simulink library "lib_accessory"  (Simulink 4.1.1)
undefined symbols (not defined in the file): acc_dcdc_eff, acc_elec_eff, acc_elec_efficiency, acc_elec_pwr, acc_mech_eff, acc_mech_pwr, acc_mech_trq, acc_sindafile, amb_tmp, cyc_mph, ess_on, fc_on, fd_ratio, gb_ratio, load_on, map_spd, max_pwr, tc_gc_to_fc_ratio, time_step, vc_idle_bool, vc_idle_spd, vinf, wh_radius
libraries: lib_accessory x47, lib_cosimulation x29, lib_outputs x11, simulink3 x4, sub_lib_models x2
(part 1 of 3)
settings Model: LastModifiedBy=abrooker  ModifiedComment=abrooker -- Fri Jun 21 11:06:39 2002 -- Version 1.443
settings Model: ModifiedHistory=|
  | abrooker -- Fri Jun 21 11:06:39 2002 -- Version 1.443
  | 
  | 
  | abrooker -- Fri Jun 21 11:06:32 2002 -- Version 1.442
  | 
  | 
  | abrooker -- Fri Jun 21 11:03:06 2002 -- Version 1.441
  | 
  | 
  | abrooker -- Fri Jun 21 08:18:53 2002 -- Version 1.440
  | 
  | 
  | abrooker -- Fri Jun 21 08:07:14 2002 -- Version 1.439
  | 
  | 
  | abrooker -- Fri Jun 21 07:53:07 2002 -- Version 1.438
  | 
  | 
  | abrooker -- Thu Jun 20 15:33:10 2002 -- Version 1.437
  | 
  | 
  | abrooker -- Thu Jun 20 15:32:18 2002 -- Version 1.436
  | 
  | 
  | mokeefe -- Wed May 22 16:23:29 2002 -- Version 1.435
  | changed SindaTransAC model to take 5 outputs
  | 
  | mokeefe -- Thu Apr 18 08:24:09 2002 -- Version 1.434
  | saving the model:
  | o "without the model browser open"
  | o with only top-level screen visible
  | o with "fit to view" enabled
  | o with "status bar" off and "toolbar" off
  | o with "prompt to update model history with each save" on
  | 
  | tmarkel -- Mon Apr 15 11:38:46 2002 -- Version 1.428
  | 
  | 
  | tmarkel -- Mon Apr 15 11:38:46 2002 -- Version 1.428
  | 
  | 
  | tmarkel -- Mon Apr 15 11:38:36 2002 -- Version 1.427
  | 
  | 
  | mokeefe -- Mon Apr 15 11:36:55 2002 -- Version 1.426
  | added acc_sindafile variable into the SindaTransAC model
  | 
  | 
  | 
  | 
  | 
  | mokeefe -- Mon Apr 15 11:30:03 2002 -- Version 1.424
  | adding a feature to the sinda fluint s-function so that user can pass in the path to their executable file (*.im) function
  | 
  | 
  | abrooker -- Thu Apr 11 17:26:32 2002 -- Version 1.423
  | added vc_idle_bool in minimum fc shaft speed for stop/start:  otherwise
  | 
  | mokeefe -- Wed Apr 03 17:17:08 2002 -- Version 1.422
  | checked the configurable sub-system option for SindaTransAC
  | 
  | abrooker -- Tue Apr 02 08:21:35 2002 -- Version 1.421
  | 
  | 
  | abrooker -- Tue Apr 02 08:16:39 2002 -- Version 1.420
  | 
  | 
  | mokeefe -- Fri Mar 29 16:21:02 2002 -- Version 1.419
  | 
  | 
  | mokeefe -- Fri Mar 29 16:18:34 2002 -- Version 1.418
  | added SindaTransAC Sinda/Fluint cosim aux. model (transient air condition modeling)
  | 
  | mokeefe -- Fri Mar 29 09:01:44 2002 -- Version 1.417
  | 
  | 
  | mokeefe -- Fri Mar 29 09:00:29 2002 -- Version 1.416
  | 
  | 
  | mokeefe -- Fri Mar 29 08:55:21 2002 -- Version 1.415
  | 
  | 
  | mokeefe -- Fri Mar 29 08:54:32 2002 -- Version 1.414
  | 
  | 
  | mokeefe -- Fri Mar 29 08:34:07 2002 -- Version 1.413
  | 
  | 
  | mokeefe -- Fri Mar 29 08:33:22 2002 -- Version 1.412
  | rearranging the library for aesthetic purposes =)
  | 
  | mokeefe -- Fri Mar 29 08:27:44 2002 -- Version 1.411
  | took out two of the mechanical accessory options that will probably not be used (the same functionality is available with the remaining blocks). These blocks moved to the development subsystem for storage.
  | 
  | abrooker -- Thu Mar 28 16:18:46 2002 -- Version 1.410
  | (mokeefe) changed the Mechanical Accessory Load Driveline Block to use memory blocks for torque and power estimation (as opposed to two calculations)
  | 
  | abrooker -- Thu Mar 28 12:33:24 2002 -- Version 1.409
  | 
  | 
  | abrooker -- Thu Mar 28 12:25:41 2002 -- Version 1.408
  | 
  | 
  | abrooker -- Thu Mar 28 12:08:36 2002 -- Version 1.407
  | 
  | 
  | abrooker -- Thu Mar 28 12:04:18 2002 -- Version 1.406
  | 
  | 
  | abrooker -- Thu Mar 28 08:53:24 2002 -- Version 1.405
  | 
  | 
  | abrooker -- Thu Mar 28 08:49:44 2002 -- Version 1.404
  | 
  | 
  | mokeefe -- Wed Mar 27 07:38:24 2002 -- Version 1.403
  | 
  | 
  | mokeefe -- Wed Mar 27 07:37:49 2002 -- Version 1.402
  | added a masked variable (acc_max_spd) to the mechanical accessory loads library
  | 
  | mokeefe -- Wed Mar 20 10:22:56 2002 -- Version 1.401
  | changed the pictures for the configurable subsystem blocks to differentiate from the driveline blocks
  | 
  | mokeefe -- Tue Mar 12 13:44:43 2002 -- Version 1.400
  | 
  | 
  | mokeefe -- Tue Mar 12 13:36:01 2002 -- Version 1.399
  | cleaned up the library and reorganized block positions
  | 
  | 
  | mokeefe -- Tue Mar 12 13:34:33 2002 -- Version 1.398
  | 
  | 
  | mokeefe -- Tue Mar 12 13:34:15 2002 -- Version 1.397
  | 
  | 
  | mokeefe -- Tue Mar 12 13:29:31 2002 -- Version 1.396
  | 
  | 
  | mokeefe -- Tue Mar 12 13:25:46 2002 -- Version 1.395
  | 
  | 
  | mokeefe -- Tue Mar 12 13:09:55 2002 -- Version 1.394
  | changed the variable mechanical loads to include a water pump
  | 
  | mokeefe -- Tue Mar 12 12:07:07 2002 -- Version 1.393
  | 
  | 
  | mokeefe -- Tue Mar 12 12:06:03 2002 -- Version 1.392
  | 
  | 
  | mokeefe -- Tue Mar 12 12:04:31 2002 -- Version 1.391
  | 
  | 
  | mokeefe -- Tue Mar 12 11:59:22 2002 -- Version 1.390
  | 
  | 
  | mokeefe -- Tue Mar 12 11:54:25 2002 -- Version 1.389
  | changing the way that data signals are recorded (especially for the variable mechanical loads blocks--see SubLibraries/variable mechanical load --simulink implementation--)
  | 
  | mokeefe -- Fri Mar 08 07:13:02 2002 -- Version 1.388
  | added the tag acc_mech_pwr_est as a global tag to Mechanical Accessory Loads v2 <acc>
  | 
  | mokeefe -- Mon Mar 04 07:28:37 2002 -- Version 1.387
  | 
  | 
  | mokeefe -- Mon Mar 04 07:27:09 2002 -- Version 1.386
  | 
  | 
  | mokeefe -- Mon Mar 04 07:24:49 2002 -- Version 1.385
  | changed the mechanical accessory torque back to a simple version
  | 
  | mokeefe -- Fri Mar 01 16:40:21 2002 -- Version 1.384
  | 
  | 
  | mokeefe -- Fri Mar 01 16:37:19 2002 -- Version 1.383
  | 
  | 
  | mokeefe -- Fri Mar 01 15:08:33 2002 -- Version 1.382
  | 
  | 
  | mokeefe -- Fri Mar 01 12:12:06 2002 -- Version 1.381
  | 
  | 
  | mokeefe -- Fri Mar 01 12:10:27 2002 -- Version 1.380
  | 
  | 
  | mokeefe -- Fri Mar 01 11:39:14 2002 -- Version 1.379
  | 
  | 
  | mokeefe -- Fri Mar 01 11:20:41 2002 -- Version 1.378
  | 
  | 
  | mokeefe -- Fri Mar 01 10:50:57 2002 -- Version 1.377
  | 
  | 
  | mokeefe -- Fri Mar 01 10:18:24 2002 -- Version 1.376
  | 
  | 
  | mokeefe -- Fri Mar 01 10:16:01 2002 -- Version 1.375
  | 
  | 
  | mokeefe -- Fri Mar 01 10:13:39 2002 -- Version 1.374
  | 
  | 
  | mokeefe -- Fri Mar 01 09:58:45 2002 -- Version 1.373
  | 
  | 
  | mokeefe -- Fri Mar 01 09:31:13 2002 -- Version 1.372
  | 
  | 
  | mokeefe -- Fri Mar 01 09:30:34 2002 -- Version 1.371
  | 
  | 
  | mokeefe -- Fri Mar 01 09:00:19 2002 -- Version 1.370
  | 
  | 
  | mokeefe -- Fri Mar 01 08:27:00 2002 -- Version 1.369
  | 
  | 
  | mokeefe -- Fri Mar 01 08:04:14 2002 -- Version 1.368
  | 
  | 
  | mokeefe -- Thu Feb 28 08:51:52 2002 -- Version 1.367
  | 
  | 
  | mokeefe -- Thu Feb 28 08:48:14 2002 -- Version 1.366
  | 
  | 
  | mokeefe -- Thu Feb 28 08:21:55 2002 -- Version 1.365
  | 
  | 
  | mokeefe -- Thu Feb 28 08:20:46 2002 -- Version 1.364
  | adding an on/off flag for auxiliary systems to account for "engine off" states
  | 
  | mokeefe -- Thu Feb 28 08:10:24 2002 -- Version 1.363
  | 
  | 
  | mokeefe -- Wed Feb 27 14:38:39 2002 -- Version 1.362
  | 
  | 
  | mokeefe -- Wed Feb 27 14:34:06 2002 -- Version 1.361
  | 
  | 
  | mokeefe -- Wed Feb 27 14:33:33 2002 -- Version 1.360
  | 
  | 
  | mokeefe -- Wed Feb 27 14:29:19 2002 -- Version 1.359
  | 
  | 
  | mokeefe -- Wed Feb 27 14:12:33 2002 -- Version 1.358
  | 
  | 
  | mokeefe -- Wed Feb 27 14:11:56 2002 -- Version 1.357
  | 
  | 
  | mokeefe -- Wed Feb 27 14:06:17 2002 -- Version 1.356
  | 
  | 
  | mokeefe -- Wed Feb 27 14:04:01 2002 -- Version 1.355
  | added a "version 2" to mechanical auxiliary loads library which has a workaround that takes in the fc_spd_est instead of fc_spd_out_a--this enables vehicles to have an exact match between ADVISOR v3.2 and v2002
  | 
  | mokeefe -- Wed Feb 27 09:55:44 2002 -- Version 1.354
  | 
  | 
  | mokeefe -- Wed Feb 27 09:53:42 2002 -- Version 1.
  | 
  | mokeefe -- Tue Feb 26 15:16:41 2002 -- Version 1.352
  | 
  | 
  | mokeefe -- Tue Feb 26 14:01:11 2002 -- Version 1.351
  | 
  | 
  | mokeefe -- Tue Feb 26 13:25:47 2002 -- Version 1.350
  | 
  | 
  | mokeefe -- Tue Feb 26 10:40:53 2002 -- Version 1.349
  | 
  | 
  | mokeefe -- Mon Feb 25 16:05:53 2002 -- Version 1.348
  | 
  | 
  | mokeefe -- Mon Feb 25 15:35:04 2002 -- Version 1.347
  | 
  | 
  | mokeefe -- Mon Feb 25 15:33:00 2002 -- Version 1.346
  | 
  | 
  | mokeefe -- Mon Feb 25 15:26:23 2002 -- Version 1.345
  | 
  | 
  | mokeefe -- Mon Feb 25 15:24:36 2002 -- Version 1.344
  | 
  | 
  | mokeefe -- Mon Feb 25 15:23:19 2002 -- Version 1.343
  | 
  | 
  | mokeefe -- Mon Feb 25 15:19:58 2002 -- Version 1.342
  | 
  | 
  | mokeefe -- Mon Feb 25 15:17:22 2002 -- Version 1.341
  | 
  | 
  | mokeefe -- Mon Feb 25 15:04:08 2002 -- Version 1.340
  | 
  | 
  | mokeefe -- Mon Feb 25 14:59:43 2002 -- Version 1.339
  | 
  | 
  | mokeefe -- Mon Feb 25 14:50:11 2002 -- Version 1.338
  | 
  | 
  | mokeefe -- Mon Feb 25 14:37:23 2002 -- Version 1.337
  | 
  | 
  | mokeefe -- Mon Feb 25 14:24:02 2002 -- Version 1.336
  | 
  | 
  | mokeefe -- Mon Feb 25 14:19:40 2002 -- Version 1.335
  | 
  | 
  | mokeefe -- Mon Feb 25 14:14:18 2002 -- Version 1.334
  | 
  | 
  | mokeefe -- Mon Feb 25 14:09:13 2002 -- Version 1.333
  | 
  | 
  | mokeefe -- Mon Feb 25 13:38:54 2002 -- Version 1.332
  | 
  | 
  | mokeefe -- Mon Feb 25 13:38:02 2002 -- Version 1.331
  | 
  | 
  | mokeefe -- Wed Feb 20 09:52:02 2002 -- Version 1.330
  | 
  | 
  | mokeefe -- Wed Feb 20 09:49:29 2002 -- Version 1.329
  | changed the acc_mech_trq_a, acc_mech_pwr_a, acc_mech_trq_r, acc_mech_pwr_r, acc_elec_pwr_a, acc_elec_pwr_r GOTO blocks to global scope.
  | 
  | mokeefe -- Wed Feb 20 09:47:28 2002 -- Version 1.328
  | 
  | 
  | mokeefe -- Wed Feb 20 09:46:46 2002 -- Version 1.327
  | 
  | 
  | mokeefe -- Wed Feb 20 07:42:37 2002 -- Version 1.326
  | 
  | 
  | mokeefe -- Wed Feb 20 07:42:12 2002 -- Version 1.325
  | 
  | 
  | mokeefe -- Wed Feb 20 07:41:46 2002 -- Version 1.324
  | 
  | 
  | mokeefe -- Tue Feb 19 16:34:31 2002 -- Version 1.323
  | 
  | 
  | mokeefe -- Tue Feb 19 16:31:37 2002 -- Version 1.322
  | 
  | 
  | mokeefe -- Tue Feb 19 16:28:38 2002 -- Version 1.321
  | changed the accessory GOTO tags to global scope in Electrical Accessory Loads
  | 
  | mokeefe -- Tue Feb 19 16:14:33 2002 -- Version 1.320
  | first release to RCS
  | 
  | mokeefe -- Tue Feb 19 16:12:28 2002 -- Version 1.319
  | 
  | 
  | mokeefe -- Tue Feb 19 16:06:11 2002 -- Version 1.318
  | 
  | 
  | mokeefe -- Tue Feb 19 16:02:32 2002 -- Version 1.317
  | 
  | 
  | mokeefe -- Tue Feb 19 15:58:43 2002 -- Version 1.316
  | 
  | 
  | mokeefe -- Tue Feb 19 15:55:41 2002 -- Version 1.315
  | 
  | 
  | mokeefe -- Tue Feb 19 15:53:46 2002 -- Version 1.314
  | 
  | 
  | mokeefe -- Tue Feb 19 15:49:12 2002 -- Version 1.313
  | 
  | 
  | mokeefe -- Tue Feb 19 15:42:48 2002 -- Version 1.312
  | 
  | 
  | mokeefe -- Tue Feb 19 15:41:05 2002 -- Version 1.311
  | 
  | 
  | mokeefe -- Tue Feb 19 15:38:40 2002 -- Version 1.310
  | 
  | 
  | mokeefe -- Tue Feb 19 15:28:06 2002 -- Version 1.309
  | 
  | 
  | mokeefe -- Tue Feb 19 15:18:02 2002 -- Version 1.308
  | 
  | 
  | mokeefe -- Tue Feb 19 14:53:21 2002 -- Version 1.307
  | 
  | 
  | mokeefe -- Tue Feb 19 14:46:24 2002 -- Version 1.306
  | 
  | 
  | mokeefe -- Tue Feb 19 14:20:08 2002 -- Version 1.305
  | 
  | 
  | mokeefe -- Tue Feb 19 14:15:36 2002 -- Version 1.304
  | 
  | 
  | mokeefe -- Tue Feb 19 13:24:42 2002 -- Version 1.303
  | 
  | 
  | mokeefe -- Tue Feb 19 13:17:05 2002 -- Version 1.302
  | 
  | 
  | mokeefe -- Tue Feb 19 13:11:20 2002 -- Version 1.301
  | 
  | 
  | mokeefe -- Tue Feb 19 11:29:38 2002 -- Version 1.300
  | 
  | 
  | mokeefe -- Tue Feb 19 11:24:45 2002 -- Version 1.299
  | adding electrical accessory block
  | 
  | 
  | mokeefe -- Tue Feb 19 10:53:36 2002 -- Version 1.298
  | 
  | 
  | mokeefe -- Tue Feb 19 10:19:54 2002 -- Version 1.297
  | added electrical accessory loads block
  | 
  | 
  | mokeefe -- Thu Feb 14 17:56:03 2002 -- Version 1.296
  | 
  | 
  | mokeefe -- Thu Feb 14 17:54:33 2002 -- Version 1.295
  | 
  | 
  | mokeefe -- Thu Feb 14 17:51:07 2002 -- Version 1.294
  | 
  | 
  | mokeefe -- Thu Feb 14 17:49:19 2002 -- Version 1.293
  | changing the way that data is "logged" to displays and scopes vs. workspace on some components that I expect will have to be used multiple times... (a workaround for now)
  | 
  | mokeefe -- Thu Feb 14 17:21:35 2002 -- Version 1.292
  | 
  | 
  | mokeefe -- Thu Feb 14 16:55:33 2002 -- Version 1.291
  | 
  | 
  | mokeefe -- Thu Feb 14 16:21:30 2002 -- Version 1.290
  | 
  | 
  | mokeefe -- Thu Feb 14 16:19:08 2002 -- Version 1.289
  | 
  | 
  | mokeefe -- Thu Feb 14 16:17:00 2002 -- Version 1.288
  | 
  | 
  | mokeefe -- Thu Feb 14 16:15:50 2002 -- Version 1.287
  | 
  | 
  | mokeefe -- Thu Feb 14 16:14:24 2002 -- Version 1.286
  | 
  | 
  | mokeefe -- Thu Feb 14 16:13:43 2002 -- Version 1.285
  | 
  | 
  | mokeefe -- Thu Feb 14 15:43:46 2002 -- Version 1.284
  | 
  | 
  | mokeefe -- Thu Feb 14 15:42:22 2002 -- Version 1.283
  | 
  | 
  | mokeefe -- Thu Feb 14 15:31:24 2002 -- Version 1.282
  | 
  | 
  | mokeefe -- Thu Feb 14 15:26:13 2002 -- Version 1.281
  | 
  | 
  | mokeefe -- Thu Feb 14 15:25:37 2002 -- Version 1.280
  | 
  | 
  | mokeefe -- Thu Feb 14 15:19:19 2002 -- Version 1.279
  | 
  | 
  | mokeefe -- Thu Feb 14 15:10:41 2002 -- Version 1.278
  | 
  | 
  | mokeefe -- Thu Feb 14 14:28:51 2002 -- Version 1.277
  | 
  | 
  | mokeefe -- Thu Feb 14 14:26:34 2002 -- Version 1.276
  | 
  | 
  | mokeefe -- Thu Feb 14 10:50:49 2002 -- Version 1.275
  | 
  | 
  | mokeefe -- Thu Feb 14 10:47:05 2002 -- Version 1.274
  | 
  | 
  | mokeefe -- Thu Feb 14 10:40:54 2002 -- Version 1.273
  | 
  | 
  | mokeefe -- Thu Feb 14 10:23:01 2002 -- Version 1.272
  | 
  | 
  | mokeefe -- Thu Feb 14 10:05:05 2002 -- Version 1.271
  | 
  | 
  | mokeefe -- Thu Feb 14 09:56:25 2002 -- Version 1.270
  | 
  | 
  | mokeefe -- Thu Feb 14 09:55:54 2002 -- Version 1.269
  | changed the "signal width" parameters of blocks such that they work correctly
  | 
  | mokeefe -- Thu Feb 14 09:54:47 2002 -- Version 1.268
  | 
  | 
  | mokeefe -- Thu Feb 14 09:51:13 2002 -- Version 1.267
  | 
  | 
  | mokeefe -- Thu Feb 14 08:58:02 2002 -- Version 1.266
  | 
  | 
  | mokeefe -- Thu Feb 14 08:39:00 2002 -- Version 1.265
  | changed the port width in alternator block back to dynamically sized
  | 
  | 
  | mokeefe -- Thu Feb 14 08:06:18 2002 -- Version 1.264
  | 
  | 
  | mokeefe -- Wed Feb 13 16:52:46 2002 -- Version 1.263
  | adding signal specification blocks to force the size of signals
  | 
  | mokeefe -- Wed Feb 13 16:52:26 2002 -- Version 1.262
  | 
  | 
  | mokeefe -- Wed Feb 13 16:46:44 2002 -- Version 1.261
  | 
  | 
  | mokeefe -- Wed Feb 13 16:31:21 2002 -- Version 1.260
  | 
  | 
  | mokeefe -- Wed Feb 13 16:30:50 2002 -- Version 1.259
  | 
  | 
  | mokeefe -- Wed Feb 13 16:25:26 2002 -- Version 1.258
  | 
  | 
  | mokeefe -- Wed Feb 13 15:56:34 2002 -- Version 1.257
  | testing
  | 
  | 
  | mokeefe -- Wed Feb 13 14:44:42 2002 -- Version 1.256
  | the accessory library

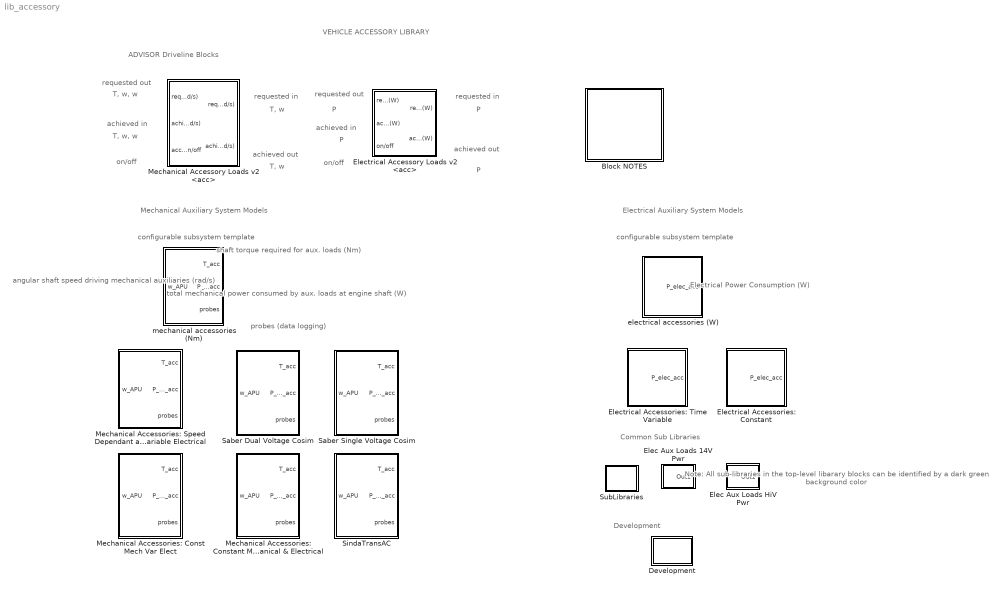
== system lib_accessory ==
  note: Common Sub Libraries
  note: Note:
      | All sub-libraries
      | in the top-level libarary
      | blocks can be identified
      | by a dark green background color
  note: VEHICLE ACCESSORY LIBRARY
  note: Mechanical Auxiliary System Models
  note: ADVISOR Driveline Blocks
  note: Electrical Auxiliary System Models
  note: configurable subsystem template
  note: total mechanical
      | power consumed by
      | aux. loads
      | at engine shaft (W)
  note: shaft torque required
      | for aux. loads (Nm)
  note: angular
      | shaft
      | speed
      | driving
      | mechanical
      | auxiliaries
      | (rad/s)
  note: configurable subsystem template
  note: requested out
  note: requested in
  note: achieved in
  note: achieved out
  note: T, w, w
  note: T, w, w
  note: T, w
  note: T, w
  note: on/off
  note: requested out
  note: achieved in
  note: P
  note: P
  note: requested in
  note: achieved out
  note: P
  note: P
  note: on/off
  note: Development
  note: probes (data logging)
  note: Electrical Power
      | Consumption (W)
  Block NOTES : Subsystem
      settings: RTWFcnNameOpts=Auto  RTWFileNameOpts=Auto
      mask Display: disp('Model\nNOTES')
  Development : Subsystem
      settings: RTWFcnNameOpts=Auto  RTWFileNameOpts=Auto
  Elec Aux Loads 14V Pwr : Subsystem
      settings: RTWFcnNameOpts=Auto  RTWFileNameOpts=Auto
  Elec Aux Loads HiV Pwr : Subsystem
      settings: RTWFcnNameOpts=Auto  RTWFileNameOpts=Auto
  Electrical Accessories: Constant : Subsystem
      settings: RTWFcnNameOpts=Auto  RTWFileNameOpts=Auto
      mask Display: image(imread('bdi_acc_elec_cs.bmp'))
  Electrical Accessories: Time Variable : Subsystem
      settings: RTWFcnNameOpts=Auto  RTWFileNameOpts=Auto
      mask Display: image(imread('bdi_acc_elec_cs.bmp'))
  Electrical Accessory Loads v2 <acc> : Subsystem  mask{load_on=1}
      mask prompts: load_on "1 to enable loads; 0 to disable"
      settings: RTWFcnNameOpts=Auto  RTWFileNameOpts=Auto
      mask Display: image(imread('bdi_acc_elec.bmp'))
  Mechanical Accessories: Const Mech Var Elect : Subsystem
      settings: RTWFcnNameOpts=Auto  RTWFileNameOpts=Auto
      mask Display: image(imread('bdi_acc_pic_cs.bmp'))
  Mechanical Accessories: Constant Mechanical & Electrical : Subsystem
      settings: RTWFcnNameOpts=Auto  RTWFileNameOpts=Auto
      mask Display: image(imread('bdi_acc_pic_cs.bmp'))
  Mechanical Accessories: Speed Dependant and Variable Electrical : Subsystem
      settings: RTWFcnNameOpts=Auto  RTWFileNameOpts=Auto
      mask Display: image(imread('bdi_acc_pic_cs.bmp'))
  Mechanical Accessory Loads v2 <acc> : Subsystem  mask{load_on=1, acc_max_spd=inf, acc_min_spd=(vc_idle_spd+eps)*vc_idle_bool, ic_mech_trq=0, ic_mech_pwr=0}
      mask prompts: load_on "Electrical Load Status: 1 on; 0 off"; acc_max_spd "maximum shaft speed for aux. (rad/s)"; acc_min_spd "minimum shaft speed for aux. (rad/s)"; ic_mech_trq "Initial Mechanical Torque of the Accessory Loads (Nm)"; ic_mech_pwr "Initial Mechanical Auxiliary Load Power (W)"
      settings: RTWFcnNameOpts=Auto  RTWFileNameOpts=Auto
      mask Display: image(imread('bdi_acc_pic.bmp'))
  Saber Dual Voltage Cosim : Subsystem
      settings: RTWFcnNameOpts=Auto  RTWFileNameOpts=Auto
      mask Display: image(imread('bdi_acc_pic_cs.bmp'))
  Saber Single Voltage Cosim : Subsystem
      settings: RTWFcnNameOpts=Auto  RTWFileNameOpts=Auto
      mask Display: image(imread('bdi_acc_pic_cs.bmp'))
  SindaTransAC : Subsystem
      settings: RTWFcnNameOpts=Auto  RTWFileNameOpts=Auto
      mask Display: image(imread('bdi_acc_pic_cs.bmp'))
  SubLibraries : Subsystem
      settings: RTWFcnNameOpts=Auto  RTWFileNameOpts=Auto
  electrical accessories (W) : Subsystem  BlockChoice=Electrical Accessories: Time Variable
      settings: TemplateBlock=self  MemberBlocks=Electrical Accessories: Constant,Electrical Accessories: Time Variable  RTWFcnNameOpts=Auto  RTWFileNameOpts=Auto
      mask Display: image(imread('bdi_acc_elec_cs.bmp'))
  mechanical accessories (Nm) : Subsystem  BlockChoice=Mechanical Accessories: Const Mech Var Elect
      settings: TemplateBlock=self  MemberBlocks=Mechanical Accessories: Const Mech Var Elect,Mechanical Accessories: Constant Mechanical & Electrical,Mechanical Accessories: Speed Dependant and Variable Electrical,Saber Dual Voltage Cosim,Saber Single Voltage Cosim,SindaTransAC  RTWFcnNameOpts=Auto  RTWFileNameOpts=Auto
      mask Display: image(imread('bdi_acc_pic_cs.bmp'))

== system lib_accessory/Block NOTES ==
  note: The accessory library defines ADVISOR driveline blocks and their submodels/subsystems having
      | to do with mechanical and electrical auxiliary loads. Note that time-variable electrical load
      | models are defined in sublib_models.mdl (a library file)
  note: Each driveline block takes in a power or torque/speed request and augments that request
      | up the driveline toward the prime mover or power generator. On the way down, the power use
      | is re-accounted such that only the driveline energy is sent. The basic assumption is that auxiliary
      | loads are satisfied first and then power is sent down the driveline. Users may wish to implement their
      | own custom control strategies if this is not the case.
  note: This library uses configurable subsystems extensively to maximize the basic interfaces and
      | isolate the things that change from the things that stay the same. Configurable subsystems
      | are added to the model by clicking on the configurable subsystem block template (outlined in blue)
      | and checking the box next to the model name you would like to add.
  note: load_on is used as a flag in the models to switch aux loads on and off
  note: "Mechanical Loads" and "Electrical Loads" are distinguised by what form of energy
      | would have to pass the boundary of the auxiliary system model to power the
      | accessory loads. For example, a mechanical load may have electrical loads and
      | an alternator built into the model. However, if shaft energy must be supplied to
      | power the mechanical load, then the load is considered a Mechanical load because
      | it requires the shaft power as an input to the auxiliary model.
      |
      | Conversely, a load that feeds off of a power bus would be termed an electrical load

== system lib_accessory/Development ==
  note: requested out
  note: requested in
  note: achieved in
  note: achieved out
  note: T, w
  note: T, w
  note: T, w
  note: T, w
  note: requested out
  note: achieved in
  note: P
  note: P
  note: requested in
  note: achieved out
  note: P
  note: P
  note: These are old models and developmental models
  note: total mechanical
      | power consumed by
      | aux. loads
      | at engine shaft (W)
  note: angular
      | shaft
      | speed
      | driving
      | mechanical
      | auxiliaries
      | (rad/s)
  note: shaft torque required
      | for aux. loads (Nm)
  note: total mechanical
      | power consumed by
      | aux. loads
      | at engine shaft (W)
  note: angular
      | shaft
      | speed
      | driving
      | mechanical
      | auxiliaries
      | (rad/s)
  note: shaft torque required
      | for aux. loads (Nm)
  Electrical Accessory Loads <acc> : Subsystem  mask{load_on=1}
      mask prompts: load_on "1 to enable loads; 0 to disable"
      settings: RTWFcnNameOpts=Auto  RTWFileNameOpts=Auto
      mask Display: image(imread('bdi_acc_elec.bmp'))
  Mechanical Accessories: Constant Load No Alternator : Subsystem
      settings: RTWFcnNameOpts=Auto  RTWFileNameOpts=Auto
      mask Display: image(imread('bdi_acc_pic_cs.bmp'))
  Mechanical Accessories: Speed Dependant No Alternator : Subsystem
      settings: RTWFcnNameOpts=Auto  RTWFileNameOpts=Auto
      mask Display: image(imread('bdi_acc_pic_cs.bmp'))
  Mechanical Accessory Loads <acc> : Subsystem  mask{load_on=1}
      mask prompts: load_on "Electrical Load Status: 1 on; 0 off"
      settings: RTWFcnNameOpts=Auto  RTWFileNameOpts=Auto
      mask Display: image(imread('bdi_acc_pic.bmp'))
  variable mechanical load : Subsystem
      settings: RTWFcnNameOpts=Auto  RTWFileNameOpts=Auto

== system lib_accessory/Elec Aux Loads 14V Pwr ==
  BrakeLights : Subsystem
      settings: RTWFcnNameOpts=Auto  RTWFileNameOpts=Auto
  Constant : Constant  Value=0
  Constant1 : Constant  Value=vinf.AuxLoadsOn
  Engine : Subsystem
      settings: RTWFcnNameOpts=Auto  RTWFileNameOpts=Auto
  ExternalLights : Subsystem
      settings: RTWFcnNameOpts=Auto  RTWFileNameOpts=Auto
  FrontHVAC : Subsystem
      settings: RTWFcnNameOpts=Auto  RTWFileNameOpts=Auto
  FrontWipers : Subsystem
      settings: RTWFcnNameOpts=Auto  RTWFileNameOpts=Auto
  HeatedSeats : Subsystem
      settings: RTWFcnNameOpts=Auto  RTWFileNameOpts=Auto
  Misc : Subsystem
      settings: RTWFcnNameOpts=Auto  RTWFileNameOpts=Auto
  RadiatorCoolingFan : Subsystem
      settings: RTWFcnNameOpts=Auto  RTWFileNameOpts=Auto
  Radio : Subsystem
      settings: RTWFcnNameOpts=Auto  RTWFileNameOpts=Auto
  RearDefrost : Subsystem
      settings: RTWFcnNameOpts=Auto  RTWFileNameOpts=Auto
  RearHVAC : Subsystem
      settings: RTWFcnNameOpts=Auto  RTWFileNameOpts=Auto
  RearWipers : Subsystem
      settings: RTWFcnNameOpts=Auto  RTWFileNameOpts=Auto
  Starter : Subsystem
      settings: RTWFcnNameOpts=Auto  RTWFileNameOpts=Auto
  Sum : Sum  Inputs=++++++++++++++  SaturateOnIntegerOverflow=on
  Switch : Switch  Threshold=.5
  TurnSignals : Subsystem
      settings: RTWFcnNameOpts=Auto  RTWFileNameOpts=Auto
  Out1 : Outport  Port=1
  wires:
  Starter/1(Out1) -> Sum/14
  BrakeLights/1(Out1) -> Sum/13
  RadiatorCoolingFan/1(Out1) -> Sum/12
  ExternalLights/1(Out1) -> Sum/11
  Engine/1(Out1) -> Sum/10
  RearHVAC/1(Out1) -> Sum/9
  FrontHVAC/1(Out1) -> Sum/8
  Misc/1(Out1) -> Sum/7
  TurnSignals/1(Out1) -> Sum/6
  FrontWipers/1(Out1) -> Sum/5
  RearWipers/1(Out1) -> Sum/4
  Radio/1(Out1) -> Sum/3
  HeatedSeats/1(Out1) -> Sum/2
  RearDefrost/1(Out1) -> Sum/1
  Constant1/1 -> Switch/2
  Constant/1 -> Switch/3
  Sum/1 -> Switch/1
  Switch/1 -> Out1/1

== system lib_accessory/Elec Aux Loads HiV Pwr ==
  Constant : Constant  Value=0
  Constant1 : Constant  Value=vinf.AuxLoadsOn
  CurrentLoad1 : Subsystem
      settings: RTWFcnNameOpts=Auto  RTWFileNameOpts=Auto
  PowerLoad1 : Subsystem
      settings: RTWFcnNameOpts=Auto  RTWFileNameOpts=Auto
  PowerLoad2 : Subsystem
      settings: RTWFcnNameOpts=Auto  RTWFileNameOpts=Auto
  PowerLoad3 : Subsystem
      settings: RTWFcnNameOpts=Auto  RTWFileNameOpts=Auto
  SpeedLoad1 : Subsystem
      settings: RTWFcnNameOpts=Auto  RTWFileNameOpts=Auto
  Starter : Subsystem
      settings: RTWFcnNameOpts=Auto  RTWFileNameOpts=Auto
  Sum : Sum  Inputs=++++++  SaturateOnIntegerOverflow=on
  Switch : Switch  Threshold=.5
  Out1 : Outport  Port=1
  wires:
  Switch/1 -> Out1/1
  Constant/1 -> Switch/3
  Constant1/1 -> Switch/2
  PowerLoad1/1(Out1) -> Sum/1
  PowerLoad2/1(Out1) -> Sum/2
  PowerLoad3/1(Out1) -> Sum/3
  CurrentLoad1/1(Out1) -> Sum/4
  SpeedLoad1/1(Out1) -> Sum/5
  Starter/1(Out1) -> Sum/6
  Sum/1 -> Switch/1

== system lib_accessory/Electrical Accessories: Constant ==
  note: (W)
  Constant : Constant  Value=load_on*acc_elec_pwr/acc_elec_efficiency
  P_elec_acc : Outport  Port=1  InitialOutput=0
  wires:
  Constant/1 -> P_elec_acc/1

== system lib_accessory/Electrical Accessories: Time Variable ==
  note: (W)
  Constant : Constant  Value=acc_elec_pwr
  Constant1 : Constant  Value=load_on
  Elec Aux Loads 14V Pwr : lib_accessory/Elec Aux Loads 14V Pwr
      settings: RTWFcnNameOpts=Auto  RTWFileNameOpts=Auto
  Elec Aux Loads HiV Pwr : lib_accessory/Elec Aux Loads HiV Pwr
      settings: RTWFcnNameOpts=Auto  RTWFileNameOpts=Auto
  Product : Product  Inputs=2  Multiplication=Element-wise(.*)  SaturateOnIntegerOverflow=on
  Sum : Sum  Inputs=+++  SaturateOnIntegerOverflow=on
  dcdc converter : Gain  Gain=1/acc_dcdc_eff  Multiplication=Element-wise(K.*u)  SaturateOnIntegerOverflow=on
  divide by eff : Gain  Gain=1/acc_elec_eff  Multiplication=Element-wise(K.*u)  SaturateOnIntegerOverflow=on
  P_elec_acc : Outport  Port=1  InitialOutput=0
  wires:
  Elec Aux Loads 14V Pwr/1 -> dcdc converter/1
  Sum/1 -> divide by eff/1
  divide by eff/1 -> Product/1
  Product/1 -> P_elec_acc/1
  Constant1/1 -> Product/2
  Constant/1 -> Sum/1
  dcdc converter/1 -> Sum/2
  Elec Aux Loads HiV Pwr/1 -> Sum/3

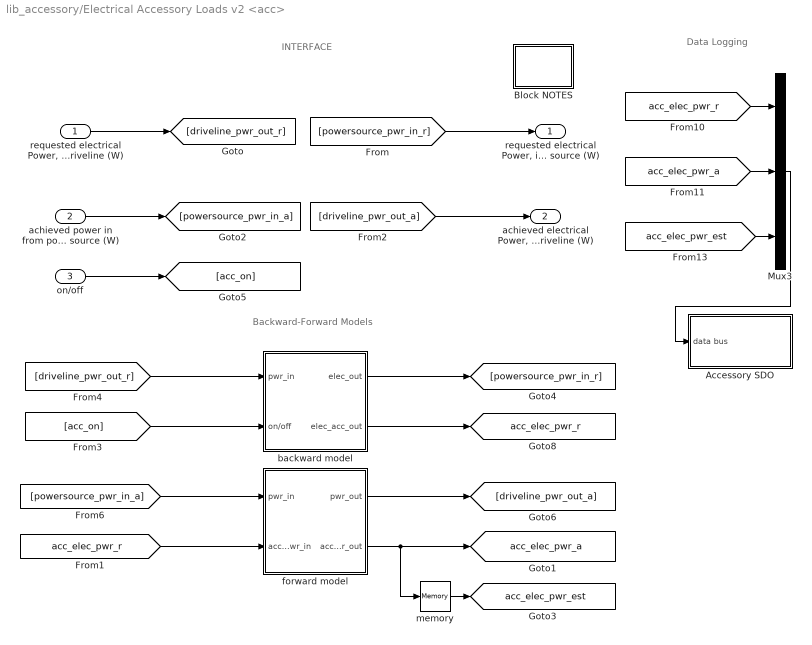
== system lib_accessory/Electrical Accessory Loads v2 <acc> ==
  note: INTERFACE
  note: Backward-Forward Models
  note: Data Logging
  "requested electrical Power, out to the driveline (W)" : Inport  Port=1  LatchInput=off
  achieved power in from power source (W) : Inport  Port=2  LatchInput=off
  on/off : Inport  Port=3  LatchInput=off
  Accessory SDO : Subsystem
      settings: RTWFcnNameOpts=Auto  RTWFileNameOpts=Auto
  Block NOTES : Subsystem
      settings: RTWFcnNameOpts=Auto  RTWFileNameOpts=Auto
      mask Display: disp('Block\nNOTES')
  Mux3 : Mux  Inputs=3
  backward model : Subsystem
      settings: RTWFcnNameOpts=Auto  RTWFileNameOpts=Auto
  forward model : Subsystem
      settings: RTWFcnNameOpts=Auto  RTWFileNameOpts=Auto
  memory : Memory  X0=acc_elec_pwr  InheritSampleTime=off
      settings: RTWStateStorageClass=Auto
  "requested electrical Power, in from the power source (W)" : Outport  Port=1
  "achieved electrical Power, out to the driveline (W)" : Outport  Port=2
  tag scope: acc_elec_pwr_a=global, acc_elec_pwr_est=global, acc_elec_pwr_r=global
  wires:
  "requested electrical Power, out to the driveline (W)"/1 -> [driveline_pwr_out_r]
  achieved power in from power source (W)/1 -> [powersource_pwr_in_a]
  [powersource_pwr_in_r] -> "requested electrical Power, in from the power source (W)"/1
  [driveline_pwr_out_a] -> "achieved electrical Power, out to the driveline (W)"/1
  [driveline_pwr_out_r] -> backward model/1(pwr_in)
  backward model/1(elec_out) -> [powersource_pwr_in_r]
  [powersource_pwr_in_a] -> forward model/1(pwr_in)
  forward model/1(pwr_out) -> [driveline_pwr_out_a]
  Mux3/1 -> Accessory SDO/1(data bus)
  backward model/2(elec_acc_out) -> [acc_elec_pwr_r]
  [acc_elec_pwr_r] -> Mux3/1
  [acc_elec_pwr_a] -> Mux3/2
  [acc_elec_pwr_est] -> Mux3/3
  [acc_elec_pwr_r] -> forward model/2(acc_pwr_in)
  forward model/2(acc_pwr_out) -> [acc_elec_pwr_a], memory/1
  memory/1 -> [acc_elec_pwr_est]
  on/off/1 -> [acc_on]
  [acc_on] -> backward model/2(on/off)

== system lib_accessory/Mechanical Accessories: Const Mech Var Elect ==
  note: engine shaft speed
  note: (Nm)
  note: (W)
  w_APU : Inport  Port=1  LatchInput=off
  Constant : Constant  Value=acc_mech_pwr
  Constant1 : Constant  Value=acc_mech_trq
  Constant2 : Constant  Value=acc_elec_pwr
  Constant3 : Constant  Value=load_on
  Elec Aux Loads 14V Pwr : lib_accessory/Elec Aux Loads 14V Pwr
      settings: RTWFcnNameOpts=Auto  RTWFileNameOpts=Auto
  Elec Aux Loads HiV Pwr : lib_accessory/Elec Aux Loads HiV Pwr
      settings: RTWFcnNameOpts=Auto  RTWFileNameOpts=Auto
  Ground : Ground
  Mux : Mux  Inputs=3
  Product : Product  Inputs=2  Multiplication=Element-wise(.*)  SaturateOnIntegerOverflow=on
  Sum1 : Sum  Inputs=+++  SaturateOnIntegerOverflow=on
  accessory mechanical torque and power calcs (Nm) : lib_accessory/SubLibraries/accessory mechanical torque and power calcs (Nm)  load_on=load_on
  dcdc converter : Gain  Gain=1/acc_dcdc_eff  Multiplication=Element-wise(K.*u)  SaturateOnIntegerOverflow=on
  T_acc : Outport  Port=1  InitialOutput=0
  P_mech_acc : Outport  Port=2  InitialOutput=0
  probes : Outport  Port=3  InitialOutput=0
  wires:
  w_APU/1 -> accessory mechanical torque and power calcs (Nm)/1
  accessory mechanical torque and power calcs (Nm)/1 -> T_acc/1
  accessory mechanical torque and power calcs (Nm)/2 -> P_mech_acc/1
  Mux/1 -> accessory mechanical torque and power calcs (Nm)/2
  Constant/1 -> Mux/1
  Constant1/1 -> Mux/2
  Product/1 -> Mux/3
  Constant3/1 -> Product/2
  Ground/1 -> probes/1
  Elec Aux Loads 14V Pwr/1 -> dcdc converter/1
  Constant2/1 -> Sum1/1
  Sum1/1 -> Product/1
  dcdc converter/1 -> Sum1/2
  Elec Aux Loads HiV Pwr/1 -> Sum1/3

== system lib_accessory/Mechanical Accessories: Constant Mechanical & Electrical ==
  note: engine shaft speed
  note: (Nm)
  note: (W)
  w_APU : Inport  Port=1  LatchInput=off
  Constant : Constant  Value=acc_mech_pwr
  Constant1 : Constant  Value=acc_mech_trq
  Constant2 : Constant  Value=acc_elec_pwr
  Constant3 : Constant  Value=load_on
  Ground : Ground
  Mux : Mux  Inputs=3
  Product : Product  Inputs=2  Multiplication=Element-wise(.*)  SaturateOnIntegerOverflow=on
  accessory mechanical torque and power calcs (Nm) : lib_accessory/SubLibraries/accessory mechanical torque and power calcs (Nm)  load_on=load_on
  T_acc : Outport  Port=1  InitialOutput=0
  P_mech_acc : Outport  Port=2  InitialOutput=0
  probes : Outport  Port=3  InitialOutput=0
  wires:
  w_APU/1 -> accessory mechanical torque and power calcs (Nm)/1
  accessory mechanical torque and power calcs (Nm)/1 -> T_acc/1
  accessory mechanical torque and power calcs (Nm)/2 -> P_mech_acc/1
  Mux/1 -> accessory mechanical torque and power calcs (Nm)/2
  Constant/1 -> Mux/1
  Constant1/1 -> Mux/2
  Constant2/1 -> Product/1
  Product/1 -> Mux/3
  Constant3/1 -> Product/2
  Ground/1 -> probes/1

== system lib_accessory/Mechanical Accessories: Speed Dependant and Variable Electrical ==
  note: engine shaft speed
  note: (Nm)
  note: (W)
  w_APU : Inport  Port=1  LatchInput=off
  Constant1 : Constant  Value=acc_elec_pwr
  Constant2 : Constant  Value=acc_mech_trq
  Constant3 : Constant  Value=load_on
  Mux : Mux  Inputs=3
  Product : Product  Inputs=2  Multiplication=Element-wise(.*)  SaturateOnIntegerOverflow=on
  accessory mechanical torque and power calcs (Nm) : lib_accessory/SubLibraries/accessory mechanical torque and power calcs (Nm)  load_on=load_on
  variable mechanical load --simulink implementation-- : lib_accessory/SubLibraries/variable mechanical load --simulink implementation--
      settings: RTWFcnNameOpts=Auto  RTWFileNameOpts=Auto
  T_acc : Outport  Port=1  InitialOutput=0
  P_mech_acc : Outport  Port=2  InitialOutput=0
  probes : Outport  Port=3  InitialOutput=0
  wires:
  w_APU/1 -> variable mechanical load --simulink implementation--/1, accessory mechanical torque and power calcs (Nm)/1
  variable mechanical load --simulink implementation--/1 -> Mux/1
  Mux/1 -> accessory mechanical torque and power calcs (Nm)/2
  accessory mechanical torque and power calcs (Nm)/1 -> T_acc/1
  accessory mechanical torque and power calcs (Nm)/2 -> P_mech_acc/1
  Constant2/1 -> Mux/2
  Constant1/1 -> Product/1
  Product/1 -> Mux/3
  Constant3/1 -> Product/2
  variable mechanical load --simulink implementation--/2 -> probes/1

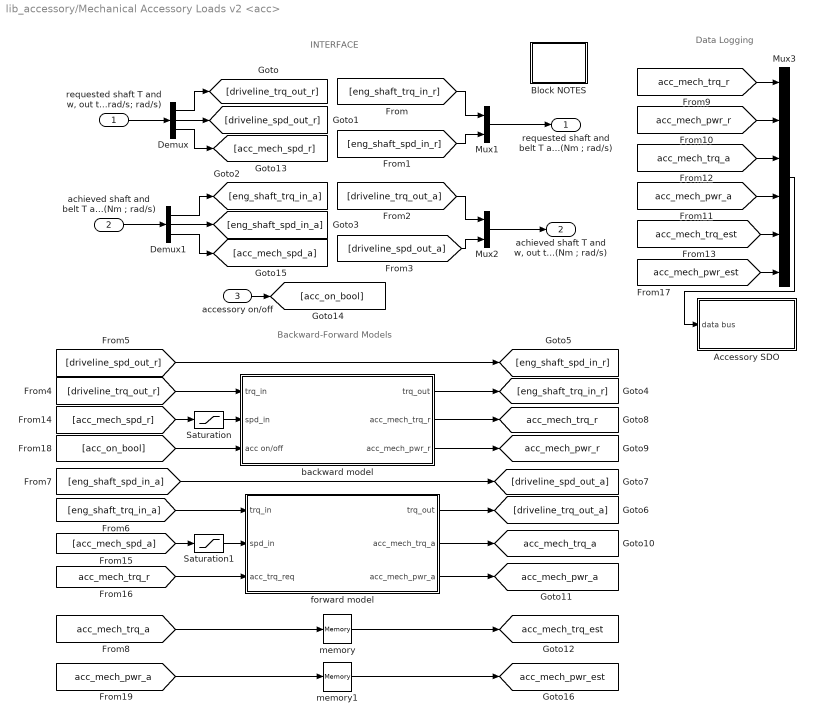
== system lib_accessory/Mechanical Accessory Loads v2 <acc> ==
  note: INTERFACE
  note: Backward-Forward Models
  note: Data Logging
  "requested shaft T and w, out to the driveline  (Nm ; rad/s; rad/s)" : Inport  Port=1  LatchInput=off
  "achieved shaft and belt T and w, in from the prime mover (Nm ; rad/s)" : Inport  Port=2  LatchInput=off
  accessory on/off : Inport  Port=3  LatchInput=off
  Accessory SDO : Subsystem
      settings: RTWFcnNameOpts=Auto  RTWFileNameOpts=Auto
  Block NOTES : Subsystem
      settings: RTWFcnNameOpts=Auto  RTWFileNameOpts=Auto
      mask Display: disp('Block\nNOTES')
  Demux : Demux  Outputs=3  BusSelectionMode=off
  Demux1 : Demux  Outputs=3  BusSelectionMode=off
  Mux1 : Mux  Inputs=2
  Mux2 : Mux  Inputs=2
  Mux3 : Mux  Inputs=6
  Saturation : Saturate  UpperLimit=acc_max_spd  LowerLimit=acc_min_spd  LinearizeAsGain=on
  Saturation1 : Saturate  UpperLimit=acc_max_spd  LowerLimit=acc_min_spd  LinearizeAsGain=on
  backward model : Subsystem
      settings: RTWFcnNameOpts=Auto  RTWFileNameOpts=Auto
  forward model : Subsystem
      settings: RTWFcnNameOpts=Auto  RTWFileNameOpts=Auto
  memory : Memory  X0=ic_mech_trq  InheritSampleTime=off
      settings: RTWStateStorageClass=Auto
  memory1 : Memory  X0=ic_mech_pwr  InheritSampleTime=off
      settings: RTWStateStorageClass=Auto
  "requested shaft and belt T and w, in from the prime mover (Nm ; rad/s)" : Outport  Port=1
  "achieved shaft T and w, out to the driveline (Nm ; rad/s)" : Outport  Port=2
  tag scope: acc_mech_pwr_a=global, acc_mech_pwr_est=global, acc_mech_pwr_r=global, acc_mech_trq_a=global, acc_mech_trq_est=global, acc_mech_trq_r=global
  wires:
  "requested shaft T and w, out to the driveline  (Nm ; rad/s; rad/s)"/1 -> Demux/1
  Demux/1 -> [driveline_trq_out_r]
  Demux/2 -> [driveline_spd_out_r]
  "achieved shaft and belt T and w, in from the prime mover (Nm ; rad/s)"/1 -> Demux1/1
  Demux1/1 -> [eng_shaft_trq_in_a]
  Demux1/2 -> [eng_shaft_spd_in_a]
  Mux1/1 -> "requested shaft and belt T and w, in from the prime mover (Nm ; rad/s)"/1
  [eng_shaft_trq_in_r] -> Mux1/1
  [eng_shaft_spd_in_r] -> Mux1/2
  Mux2/1 -> "achieved shaft T and w, out to the driveline (Nm ; rad/s)"/1
  [driveline_trq_out_a] -> Mux2/1
  [driveline_spd_out_a] -> Mux2/2
  backward model/2(acc_mech_trq_r) -> [acc_mech_trq_r]
  backward model/3(acc_mech_pwr_r) -> [acc_mech_pwr_r]
  [driveline_trq_out_r] -> backward model/1(trq_in)
  backward model/1(trq_out) -> [eng_shaft_trq_in_r]
  [acc_mech_trq_r] -> Mux3/1
  [acc_mech_pwr_r] -> Mux3/2
  Mux3/1 -> Accessory SDO/1(data bus)
  [acc_mech_trq_est] -> Mux3/5
  [driveline_spd_out_r] -> [eng_shaft_spd_in_r]
  [eng_shaft_spd_in_a] -> [driveline_spd_out_a]
  [acc_mech_trq_a] -> Mux3/3
  [acc_mech_pwr_a] -> Mux3/4
  [eng_shaft_trq_in_a] -> forward model/1(trq_in)
  accessory on/off/1 -> [acc_on_bool]
  [acc_on_bool] -> backward model/3(acc on/off)
  forward model/1(trq_out) -> [driveline_trq_out_a]
  forward model/2(acc_mech_trq_a) -> [acc_mech_trq_a]
  forward model/3(acc_mech_pwr_a) -> [acc_mech_pwr_a]
  [acc_mech_spd_a] -> Saturation1/1
  Saturation1/1 -> forward model/2(spd_in)
  [acc_mech_spd_r] -> Saturation/1
  Saturation/1 -> backward model/2(spd_in)
  [acc_mech_trq_r] -> forward model/3(acc_trq_req)
  Demux1/3 -> [acc_mech_spd_a]
  Demux/3 -> [acc_mech_spd_r]
  [acc_mech_pwr_est] -> Mux3/6
  memory/1 -> [acc_mech_trq_est]
  memory1/1 -> [acc_mech_pwr_est]
  [acc_mech_trq_a] -> memory/1
  [acc_mech_pwr_a] -> memory1/1

== system lib_accessory/Saber Dual Voltage Cosim ==
  note: (Nm)
  w_APU : Inport  Port=1  LatchInput=off
  Ground : Ground
  saber dv acc : Subsystem
      settings: RTWFcnNameOpts=Auto  RTWFileNameOpts=Auto
  T_acc : Outport  Port=1  InitialOutput=0
  P_mech_acc : Outport  Port=2  InitialOutput=0
  probes : Outport  Port=3  InitialOutput=0
  wires:
  Ground/1 -> probes/1
  saber dv acc/1(T_acc) -> T_acc/1
  saber dv acc/2(P_acc) -> P_mech_acc/1
  w_APU/1 -> saber dv acc/1(w_APU)

== system lib_accessory/Saber Single Voltage Cosim ==
  note: (Nm)
  w_APU : Inport  Port=1  LatchInput=off
  Ground : Ground
  saber sv acc : Subsystem
      settings: RTWFcnNameOpts=Auto  RTWFileNameOpts=Auto
  T_acc : Outport  Port=1  InitialOutput=0
  P_mech_acc : Outport  Port=2  InitialOutput=0
  probes : Outport  Port=3  InitialOutput=0
  wires:
  w_APU/1 -> saber sv acc/1(w_APU)
  saber sv acc/2(P_acc) -> P_mech_acc/1
  saber sv acc/1(T_acc) -> T_acc/1
  Ground/1 -> probes/1

== system lib_accessory/SindaTransAC ==
  note: (Nm)
  w_APU : Inport  Port=1  LatchInput=off
  Ground : Ground
  accessories (Nm) : Subsystem  mask{sindafile=acc_sindafile}
      mask prompts: sindafile "Path to Sinda\Fluint *.im file"
      mask init:
      | disp(['Sinda Path is ', sindafile])
      settings: RTWFcnNameOpts=Auto  RTWFileNameOpts=Auto
  T_acc : Outport  Port=1  InitialOutput=0
  P_mech_acc : Outport  Port=2  InitialOutput=0
  probes : Outport  Port=3  InitialOutput=0
  wires:
  Ground/1 -> probes/1
  accessories (Nm)/1(T_acc) -> T_acc/1
  accessories (Nm)/2(P_acc) -> P_mech_acc/1
  w_APU/1 -> accessories (Nm)/1(w_APU)

== system lib_accessory/SubLibraries ==
  note: Conventional Mechanical
      | Auxiliary Load System
  note: duty cycle (1=full on, 0=off)
  note: required power (W)
  note: Auxiliary Device:
      | Power as a function of
      | * Instantaneous Shaft Speed (rad/s) and
      | * Time Dependant (Normalized) Load (i.e., duty cycle)
  note: shaft speed (rad/s)
  note: time (s)
  note: Auxiliary Device
      | Models
  note: Auxiliary Device:
      | Power as a function of
      | * Instantaneous Shaft Speed (rad/s) and
      | * Instantaneous Load (W)
  note: ----------------------------------------------------------------------------------
  note: shaft speed (rad/s)
  note: load on device (W)
  note: required power (W)
  note: m-file lookup
  note: ----------------------------------------------------------------------------------
  note: Auxiliary Device:
      | Power as a function of
      | * Instantaneous Shaft Speed (rad/s) and
      | * Time Dependant (Normalized) Load (i.e., duty cycle)
  note: Simulink Implementation
  note: shaft speed (rad/s)
  note: time (s)
  note: duty cycle (1=full on, 0=off)
  note: required power (W)
  note: ----------------------------------------------------------------------------------
  note: Simulink Implementation
  note: Auxiliary Device:
      | Power as a function of
      | * Instantaneous Shaft Speed (rad/s) and
      | * Time Dependant (Normalized) Load (i.e., duty cycle)
  note: Data Loggers
  Shaft Speed and Actual Load Auxiliary Device : Subsystem  mask{conv_eff=, pwr_func=}
      mask prompts: conv_eff "Load Constant Conversion Efficiency (decimal 0<=eff<=1)"; pwr_func "Variable holding string of Power Function Name"
      settings: RTWFcnNameOpts=Auto  RTWFileNameOpts=Auto
  Shaft Speed and Actual Load Auxiliary Device--lookuptable : Subsystem  mask{conv_eff=, fname=}
      mask prompts: conv_eff "Load Constant Conversion Efficiency (decimal 0<=eff<=1)"; fname "Initialization M-File"
      mask init:
      | eval(fname);
      | maxSpd=max(map_spd);
      | minSpd=min(map_spd);
      settings: RTWFcnNameOpts=Auto  RTWFileNameOpts=Auto
  Shaft Speed and Time Loaded Auxiliary Device : Subsystem  mask{acc_duty=, pwr_func=}
      mask prompts: acc_duty "Accessory duty cycle vs. time (2 Col: [time, duty])"; pwr_func "Variable holding string of Power Function Name"
      settings: RTWFcnNameOpts=Auto  RTWFileNameOpts=Auto
  Shaft Speed and Time Loaded Auxiliary Device--lookuptable : Subsystem  mask{fname=, acc_duty=}
      mask prompts: fname "Initialization M-File"; acc_duty "Accessory Duty Cycle (1st Col is time, 2nd Column is load fraction)"
      mask init:
      | eval(fname); % load the script function
      | maxSpd=max(map_spd);
      | minSpd=min(map_spd);
      settings: RTWFcnNameOpts=Auto  RTWFileNameOpts=Auto
      mask Help:
      | <p>This block must contain a variable of the string of an m-file for initialization:</p>
      | 
      | <ul>
      | <li>e.g., 'myMfile' or fileName (where fileName='myMfile')</li>
      | </ul>
      | 
      | <p>The initialization m-file must contain the variables:
      | <ol>
      | <li>map_spd</li>, <li>map_load</li>, and <li>pwr_map</li>
      | </ol>
      | 
      | <p>In addition, the user must specify a matrix with the auxiliary duty cycle. This matrix is a two column matrix with time values in the first column and load fraction in the second column. Load fraction is a value from 0 to 1 which tells weather a device is "full off" "full on" or somewhere in between.</p>
      | 
      | <p>created 7 February 2002 by mpo at NREL</p>
  accessory mechanical torque and power calcs (Nm) : Subsystem  mask{load_on=load_on}
      mask prompts: load_on "FLAG: (1= don't use acc_elec_pwr; 0= use acc_elec_pwr here)"
      settings: RTWFcnNameOpts=Auto  RTWFileNameOpts=Auto
  accessory mechanical torque and power calcs  (Nm) --elec hybrid : Subsystem
      settings: RTWFcnNameOpts=Auto  RTWFileNameOpts=Auto
  data logging probes dummy : Subsystem
      settings: RTWFcnNameOpts=Auto  RTWFileNameOpts=Auto
  data logging probes for conventional mechanical loads : Subsystem
      settings: RTWFcnNameOpts=Auto  RTWFileNameOpts=Auto
  data probes : Subsystem  BlockChoice=data logging probes for conventional mechanical loads
      settings: TemplateBlock=self  MemberBlocks=data logging probes dummy,data logging probes for conventional mechanical loads  RTWFcnNameOpts=Auto  RTWFileNameOpts=Auto
  electrical power logging : Subsystem  mask{eff=acc_mech_eff}
      mask prompts: eff "efficiency of accessory systems (decimal)"
      settings: RTWFcnNameOpts=Auto  RTWFileNameOpts=Auto
  mechanical power logging : Subsystem  mask{eff=acc_mech_eff}
      mask prompts: eff "efficiency of accessory systems (decimal)"
      settings: RTWFcnNameOpts=Auto  RTWFileNameOpts=Auto
  variable mechanical load --simulink implementation-- : Subsystem
      settings: RTWFcnNameOpts=Auto  RTWFileNameOpts=Auto
  variable mechanical load --simulink implementation-- no alternator : Subsystem
      settings: RTWFcnNameOpts=Auto  RTWFileNameOpts=Auto

== system lib_accessory/electrical accessories (W) ==
  Electrical Accessories: Time Variable : lib_accessory/Electrical Accessories: Time Variable
  P_elec_acc : Outport  Port=1
  wires:
  Electrical Accessories: Time Variable/1 -> P_elec_acc/1

== system lib_accessory/mechanical accessories (Nm) ==
  w_APU : Inport  Port=1  LatchInput=off
  Mechanical Accessories: Const Mech Var Elect : lib_accessory/Mechanical Accessories: Const Mech Var Elect
  T_acc : Outport  Port=1
  P_mech_acc : Outport  Port=2
  probes : Outport  Port=3
  wires:
  w_APU/1 -> Mechanical Accessories: Const Mech Var Elect/1
  Mechanical Accessories: Const Mech Var Elect/1 -> T_acc/1
  Mechanical Accessories: Const Mech Var Elect/2 -> P_mech_acc/1
  Mechanical Accessories: Const Mech Var Elect/3 -> probes/1

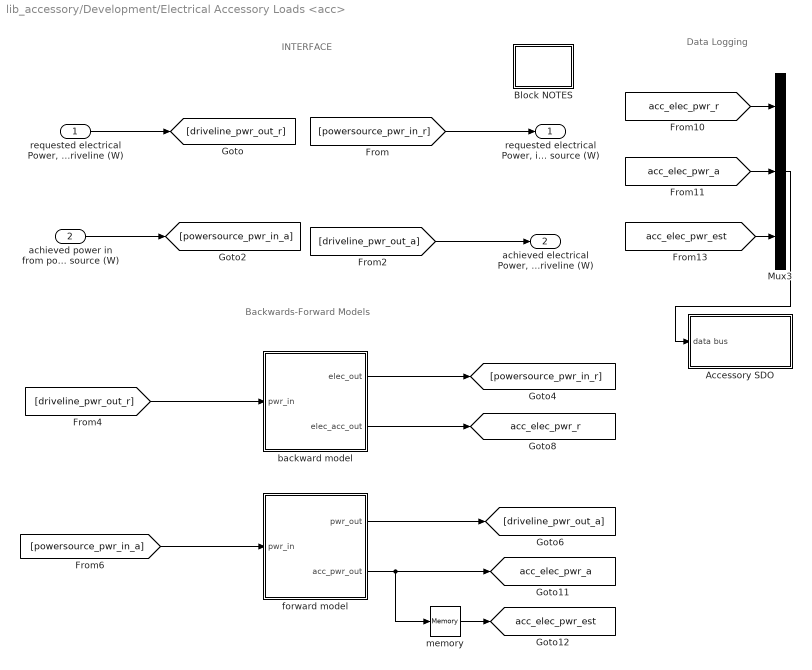
== system lib_accessory/Development/Electrical Accessory Loads <acc> ==
  note: INTERFACE
  note: Backwards-Forward Models
  note: Data Logging
  "requested electrical Power, out to the driveline (W)" : Inport  Port=1  LatchInput=off
  achieved power in from power source (W) : Inport  Port=2  LatchInput=off
  Accessory SDO : Subsystem
      settings: RTWFcnNameOpts=Auto  RTWFileNameOpts=Auto
  Block NOTES : Subsystem
      settings: RTWFcnNameOpts=Auto  RTWFileNameOpts=Auto
      mask Display: disp('Block\nNOTES')
  Mux3 : Mux  Inputs=3
  backward model : Subsystem
      settings: RTWFcnNameOpts=Auto  RTWFileNameOpts=Auto
  forward model : Subsystem
      settings: RTWFcnNameOpts=Auto  RTWFileNameOpts=Auto
  memory : Memory  X0=acc_elec_pwr  InheritSampleTime=off
      settings: RTWStateStorageClass=Auto
  "requested electrical Power, in from the power source (W)" : Outport  Port=1
  "achieved electrical Power, out to the driveline (W)" : Outport  Port=2
  tag scope: acc_elec_pwr_a=global, acc_elec_pwr_est=global, acc_elec_pwr_r=global
  wires:
  "requested electrical Power, out to the driveline (W)"/1 -> [driveline_pwr_out_r]
  achieved power in from power source (W)/1 -> [powersource_pwr_in_a]
  [powersource_pwr_in_r] -> "requested electrical Power, in from the power source (W)"/1
  [driveline_pwr_out_a] -> "achieved electrical Power, out to the driveline (W)"/1
  [driveline_pwr_out_r] -> backward model/1(pwr_in)
  backward model/1(elec_out) -> [powersource_pwr_in_r]
  [powersource_pwr_in_a] -> forward model/1(pwr_in)
  forward model/1(pwr_out) -> [driveline_pwr_out_a]
  forward model/2(acc_pwr_out) -> [acc_elec_pwr_a], memory/1
  Mux3/1 -> Accessory SDO/1(data bus)
  backward model/2(elec_acc_out) -> [acc_elec_pwr_r]
  memory/1 -> [acc_elec_pwr_est]
  [acc_elec_pwr_r] -> Mux3/1
  [acc_elec_pwr_a] -> Mux3/2
  [acc_elec_pwr_est] -> Mux3/3

== system lib_accessory/Development/Mechanical Accessories: Constant Load No Alternator ==
  note: engine shaft speed
  note: (Nm)
  note: (W)
  note: electric loads assumed to be handled elsewhere
  w_APU : Inport  Port=1  LatchInput=off
  Constant1 : Constant  Value=0
  Constant2 : Constant  Value=acc_mech_trq
  Constant3 : Constant  Value=acc_mech_pwr
  Ground : Ground
  Mux : Mux  Inputs=3
  accessory mechanical torque and power calcs (Nm) : lib_accessory/SubLibraries/accessory mechanical torque and power calcs (Nm)  load_on=load_on
  T_acc : Outport  Port=1  InitialOutput=0
  P_mech_acc : Outport  Port=2  InitialOutput=0
  probes : Outport  Port=3  InitialOutput=0
  wires:
  w_APU/1 -> accessory mechanical torque and power calcs (Nm)/1
  accessory mechanical torque and power calcs (Nm)/1 -> T_acc/1
  accessory mechanical torque and power calcs (Nm)/2 -> P_mech_acc/1
  Mux/1 -> accessory mechanical torque and power calcs (Nm)/2
  Constant2/1 -> Mux/2
  Constant1/1 -> Mux/3
  Constant3/1 -> Mux/1
  Ground/1 -> probes/1

== system lib_accessory/Development/Mechanical Accessories: Speed Dependant No Alternator ==
  note: engine shaft speed
  note: (Nm)
  note: (W)
  note: electrical loads are assumed to be handled elsewhere
  w_APU : Inport  Port=1  LatchInput=off
  Constant1 : Constant  Value=0
  Constant2 : Constant  Value=acc_mech_trq
  Mux : Mux  Inputs=3
  accessory mechanical torque and power calcs (Nm) : lib_accessory/SubLibraries/accessory mechanical torque and power calcs (Nm)  load_on=load_on
  variable mechanical load --simulink implementation-- no alternator : lib_accessory/SubLibraries/variable mechanical load --simulink implementation-- no alternator
      settings: RTWFcnNameOpts=Auto  RTWFileNameOpts=Auto
  T_acc : Outport  Port=1  InitialOutput=0
  P_mech_acc : Outport  Port=2  InitialOutput=0
  probes : Outport  Port=3  InitialOutput=0
  wires:
  w_APU/1 -> variable mechanical load --simulink implementation-- no alternator/1, accessory mechanical torque and power calcs (Nm)/1
  accessory mechanical torque and power calcs (Nm)/1 -> T_acc/1
  accessory mechanical torque and power calcs (Nm)/2 -> P_mech_acc/1
  Mux/1 -> accessory mechanical torque and power calcs (Nm)/2
  Constant2/1 -> Mux/2
  Constant1/1 -> Mux/3
  variable mechanical load --simulink implementation-- no alternator/1 -> Mux/1
  variable mechanical load --simulink implementation-- no alternator/2 -> probes/1
